simulink model "sensor_model"  (R2021a)
settings: Solver=VariableStepAuto  StartTime=0.0  StopTime=10.0  RelTol=1e-3
values from neighbouring files (symbols this model uses):
  CG = [0, 0, 0]    [constants.m]    (also in global_config.m)
  g = [0,0,-9.81]    [constants.m]    (also in global_config.m; velocity_and_forces_Jaden.m = [ q+w ; q*w ])
libraries: aerolibnav x2
settings Model: Creator=Nabil  LastModifiedBy=Nabil

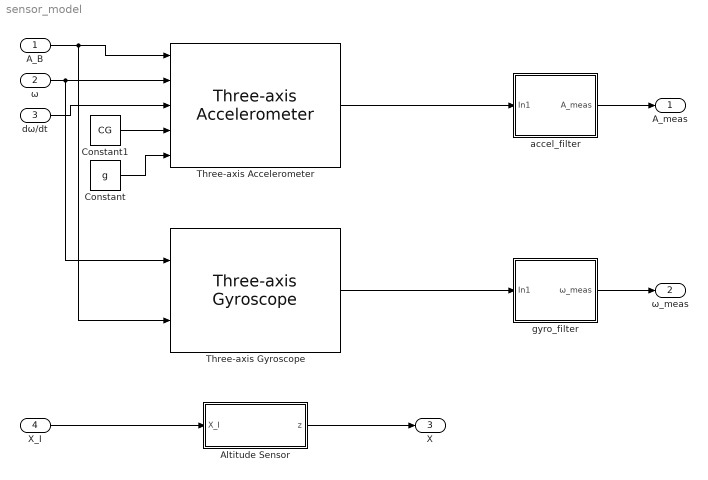
== system sensor_model ==
  A_B : Inport
  ω : Inport  Port=2
  dω/dt : Inport  Port=3
  X_I : Inport  Port=4  PortDimensions=3
  Altitude Sensor : Subsystem
  Constant : Constant  Value=g
  Constant1 : Constant  Value=CG
  Three-axis Accelerometer : aerolibnav/Three-axis Accelerometer  units=Metric (MKS)  acc=[0 0 0]  gtype=on  dtype_a=on  w_a=190  z_a=0.707  a_sf_cc=[1 0 0; 0 1 0; 0 0 1]  a_bias=[0 0 0]  a_Ts=0  a_rand=on  a_seeds=[23093 23094 23095]  a_pow=[0.001 0.001 0.001]  a_sat="[-inf  -inf  -inf  inf inf inf]"
      settings: SourceProductBaseCode=AE
  Three-axis Gyroscope : aerolibnav/Three-axis Gyroscope  dtype_g=on  w_g=190  z_g=0.707  g_sf_cc=[1 0 0; 0 1 0; 0 0 1]  g_bias=[0 0 0]  g_sen=[0 0 0]  g_Ts=0  g_rand=on  g_seeds=[23093 23094 23095]  g_pow=[0.0001 0.0001 0.0001]  g_sat="[-inf  -inf  -inf  inf inf inf]"
      settings: SourceProductBaseCode=AE
  accel_filter : Subsystem
  gyro_filter : Subsystem
  A_meas : Outport
  ω_meas : Outport  Port=2
  X : Outport  Port=3  PortDimensions=3
  wires:
  gyro_filter/1(ω_meas) -> ω_meas/1
  ω/1 -> Three-axis Gyroscope/1, Three-axis Accelerometer/2
  X_I/1 -> Altitude Sensor/1(X_I)
  Three-axis Gyroscope/1 -> gyro_filter/1(In1)
  Constant1/1 -> Three-axis Accelerometer/4
  accel_filter/1(A_meas) -> A_meas/1
  dω/dt/1 -> Three-axis Accelerometer/3
  Altitude Sensor/1(z) -> X/1
  A_B/1 -> Three-axis Gyroscope/2, Three-axis Accelerometer/1
  Three-axis Accelerometer/1 -> accel_filter/1(In1)
  Constant/1 -> Three-axis Accelerometer/5

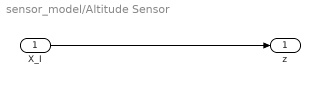
== system sensor_model/Altitude Sensor ==
  X_I : Inport
  z : Outport
  wires:
  X_I/1 -> z/1

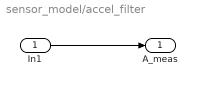
== system sensor_model/accel_filter ==
  In1 : Inport
  A_meas : Outport
  wires:
  In1/1 -> A_meas/1

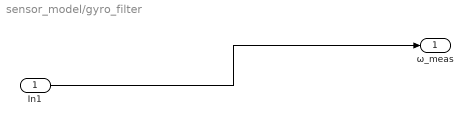
== system sensor_model/gyro_filter ==
  In1 : Inport
  ω_meas : Outport
  wires:
  In1/1 -> ω_meas/1
